simulink model "QEKF_"  (R2018a)
settings: Solver=VariableStepAuto  StartTime=0.0  StopTime=10.0  RelTol=1e-3
PreLoadFcn:
  | modelDir = fileparts(get_param(bdroot, 'FileName'));
  | addpath(fullfile(modelDir,'../../Parameters'));
  | addpath(fullfile(modelDir,'../../Estimators/QEKF'));
  | 
  | Constants_Kugle
  | Constants_nominal
  | Parameters_Estimators
  | Parameters_Simulation
InitFcn:
  | Constants_Kugle
  | Constants_nominal
  | Parameters_Estimators
  | Parameters_Simulation
undefined symbols (not defined in the file or in its folder): AccelerometerVibration_CovarianceVaryFactor, AccelerometerVibration_DetectionEnabled, AccelerometerVibration_MaxVaryFactor, AccelerometerVibration_NormLPFtau, constants_nominal, cov_acc, cov_gyro, est_q_init, EstimateBias, GyroscopeTrustFactor, NormalizeAccelerometer, QEKF_P_init_diagonal, SensorDrivenQEKF, sigma2_bias, sigma2_heading, sigma2_omega, Ts, UseHeadingEstimateFromXsensIMU
libraries: qlib x1
settings Model: Creator=Thomas  LastModifiedBy=Thomas

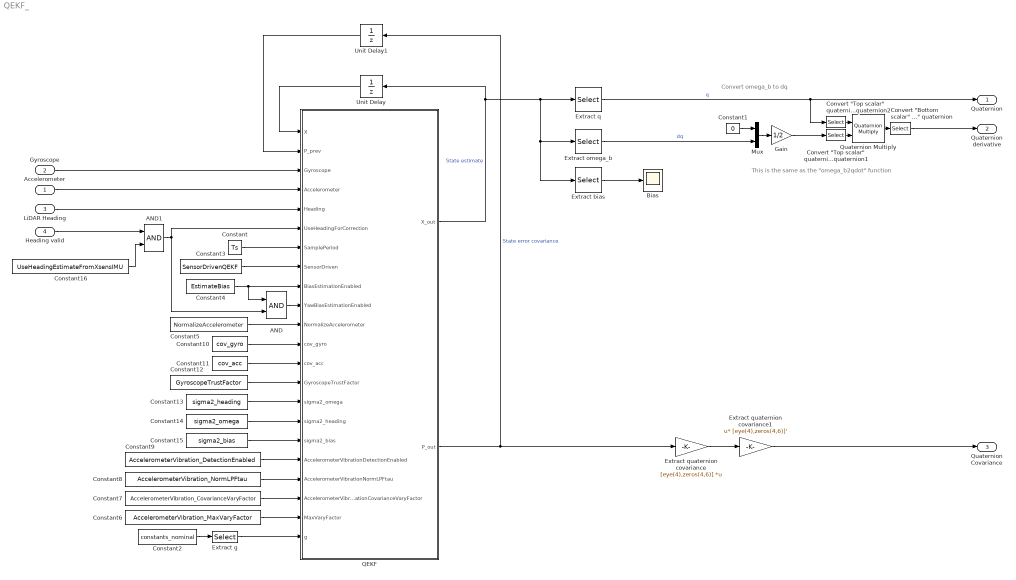
== system QEKF_ ==
  note: This is the same as the "omega_b2qdot" function
  note: Convert omega_b to dq
  Accelerometer : Inport
  Gyroscope : Inport  Port=2
  LiDAR Heading : Inport  Port=3
  Heading valid : Inport  Port=4
  AND : Logic  IconShape=distinctive  AllPortsSameDT=off  OutDataTypeStr=boolean
  AND1 : Logic  IconShape=distinctive  AllPortsSameDT=off  OutDataTypeStr=boolean
  Bias : Scope
  Constant : Constant  Value=Ts
  Constant1 : Constant  Value=0
  Constant10 : Constant  Value=cov_gyro
  Constant11 : Constant  Value=cov_acc
  Constant12 : Constant  Value=GyroscopeTrustFactor
  Constant13 : Constant  Value=sigma2_heading
  Constant14 : Constant  Value=sigma2_omega
  Constant15 : Constant  Value=sigma2_bias
  Constant16 : Constant  Value=UseHeadingEstimateFromXsensIMU
  Constant2 : Constant  Value=constants_nominal
  Constant3 : Constant  Value=SensorDrivenQEKF
  Constant4 : Constant  Value=EstimateBias
  Constant5 : Constant  Value=NormalizeAccelerometer
  Constant6 : Constant  Value=AccelerometerVibration_MaxVaryFactor
  Constant7 : Constant  Value=AccelerometerVibration_CovarianceVaryFactor
  Constant8 : Constant  Value=AccelerometerVibration_NormLPFtau
  Constant9 : Constant  Value=AccelerometerVibration_DetectionEnabled
  "Convert \"Bottom scalar\" quaternion to \"Top scalar\" quaternion" : Selector  InputPortWidth=4  IndexOptions=Index vector (dialog)  Indices=[4 1 2 3]  OutputSizes=1
  "Convert \"Top scalar\" quaternion to \"Bottom scalar\" quaternion1" : Selector  InputPortWidth=4  IndexOptions=Index vector (dialog)  Indices=[2 3 4 1]  OutputSizes=1
  "Convert \"Top scalar\" quaternion to \"Bottom scalar\" quaternion2" : Selector  InputPortWidth=4  IndexOptions=Index vector (dialog)  Indices=[2 3 4 1]  OutputSizes=1
  Extract bias : Selector  InputPortWidth=10  IndexOptions=Index vector (dialog)  Indices=[8 9 10]  OutputSizes=1
  Extract g : Selector  InputPortWidth=13  IndexOptions=Index vector (dialog)  Indices=[13]  OutputSizes=1
  Extract omega_b : Selector  InputPortWidth=10  IndexOptions=Index vector (dialog)  Indices=[5 6 7]  OutputSizes=1
  Extract q : Selector  InputPortWidth=10  IndexOptions=Index vector (dialog)  Indices=[1 2 3 4]  OutputSizes=1
  Extract quaternion covariance : Gain  Gain=[eye(4),zeros(4,6)]  Multiplication=Matrix(K*u)
  Extract quaternion covariance1 : Gain  Gain=[eye(4),zeros(4,6)]'  Multiplication=Matrix(u*K)
  Gain : Gain  Gain=1/2
  Mux : Mux  Inputs=2
  QEKF : MATLAB Function  TreatAsAtomicUnit=on
  Quaternion Multiply : qlib/Quaternion Multiply
  Unit Delay : UnitDelay  InitialCondition=[est_q_init; zeros(3,1); zeros(3,1)]  SampleTime=Ts
  Unit Delay1 : UnitDelay  InitialCondition=diag(QEKF_P_init_diagonal)  SampleTime=Ts
  Quaternion : Outport
  Quaternion derivative : Outport  Port=2
  Quaternion Covariance : Outport  Port=3
  wires:
  LiDAR Heading/1 -> QEKF/5(Heading)
  Gyroscope/1 -> QEKF/3(Gyroscope)
  Unit Delay1/1 -> QEKF/2(P_prev)
  Extract g/1 -> QEKF/22(g)
  QEKF/1(X_out) -> Unit Delay/1, Extract omega_b/1, Extract bias/1, Extract q/1  "State estimate"
  Extract bias/1 -> Bias/1
  Unit Delay/1 -> QEKF/1(X)
  Constant/1 -> QEKF/7(SamplePeriod)
  Accelerometer/1 -> QEKF/4(Accelerometer)
  AND1/1 -> QEKF/6(UseHeadingForCorrection), AND/2
  Constant1/1 -> Mux/1
  Extract omega_b/1 -> Mux/2  "dq"
  Mux/1 -> Gain/1
  Extract q/1 -> Quaternion/1, "Convert \"Top scalar\" quaternion to \"Bottom scalar\" quaternion2"/1  "q"
  "Convert \"Top scalar\" quaternion to \"Bottom scalar\" quaternion2"/1 -> Quaternion Multiply/1
  "Convert \"Top scalar\" quaternion to \"Bottom scalar\" quaternion1"/1 -> Quaternion Multiply/2
  Gain/1 -> "Convert \"Top scalar\" quaternion to \"Bottom scalar\" quaternion1"/1
  Quaternion Multiply/1 -> "Convert \"Bottom scalar\" quaternion to \"Top scalar\" quaternion"/1
  "Convert \"Bottom scalar\" quaternion to \"Top scalar\" quaternion"/1 -> Quaternion derivative/1
  Constant3/1 -> QEKF/8(SensorDriven)
  Constant4/1 -> AND/1, QEKF/9(BiasEstimationEnabled)
  AND/1 -> QEKF/10(YawBiasEstimationEnabled)
  Constant5/1 -> QEKF/11(NormalizeAccelerometer)
  Constant9/1 -> QEKF/18(AccelerometerVibrationDetectionEnabled)
  Constant8/1 -> QEKF/19(AccelerometerVibrationNormLPFtau)
  Constant7/1 -> QEKF/20(AccelerometerVibrationCovarianceVaryFactor)
  Constant6/1 -> QEKF/21(MaxVaryFactor)
  Constant10/1 -> QEKF/12(cov_gyro)
  Constant11/1 -> QEKF/13(cov_acc)
  Constant12/1 -> QEKF/14(GyroscopeTrustFactor)
  Constant13/1 -> QEKF/15(sigma2_omega)
  Constant14/1 -> QEKF/16(sigma2_heading)
  Constant15/1 -> QEKF/17(sigma2_bias)
  Constant16/1 -> AND1/2
  Heading valid/1 -> AND1/1
  Constant2/1 -> Extract g/1
  Extract quaternion covariance1/1 -> Quaternion Covariance/1
  QEKF/2(P_out) -> Extract quaternion covariance/1, Unit Delay1/1  "State error covariance"
  Extract quaternion covariance/1 -> Extract quaternion covariance1/1

== matlab function QEKF_/QEKF ==
  data: X input size=10; P_prev input size=[10,10]; X_out output size=10; Gyroscope input size=3; Accelerometer input size=3; Heading input size=1; UseHeadingForCorrection input boolean; P_out output size=[10,10]; SamplePeriod input; SensorDriven input; BiasEstimationEnabled input; YawBiasEstimationEnabled input; NormalizeAccelerometer input; cov_gyro input; cov_acc input; GyroscopeTrustFactor input; sigma2_omega input; sigma2_heading input; sigma2_bias input; AccelerometerVibrationDetectionEnabled input; AccelerometerVibrationNormLPFtau input; AccelerometerVibrationCovarianceVaryFactor input; MaxVaryFactor input; g input
function [X_out, P_out] = QEKF_(X, P_prev, Gyroscope, Accelerometer, Heading, UseHeadingForCorrection, SamplePeriod, SensorDriven, BiasEstimationEnabled, YawBiasEstimationEnabled, NormalizeAccelerometer, cov_gyro, cov_acc, GyroscopeTrustFactor, sigma2_omega, sigma2_heading, sigma2_bias, AccelerometerVibrationDetectionEnabled, AccelerometerVibrationNormLPFtau, AccelerometerVibrationCovarianceVaryFactor, MaxVaryFactor, g)
    [X_out_, P_out_] = QEKF(single(X), single(P_prev), single(Gyroscope), single(Accelerometer), single(Heading), UseHeadingForCorrection, single(SamplePeriod), SensorDriven, BiasEstimationEnabled, YawBiasEstimationEnabled, NormalizeAccelerometer, single(cov_gyro), single(cov_acc), single(GyroscopeTrustFactor), single(sigma2_omega), single(sigma2_heading), single(sigma2_bias), AccelerometerVibrationDetectionEnabled, single(AccelerometerVibrationNormLPFtau), single(AccelerometerVibrationCovarianceVaryFactor), single(MaxVaryFactor), single(g));
    X_out = double(X_out_);
    P_out = double(P_out_);
end
